simulink model "Z_Feedback_ROS"  (R2022b)
settings: Solver=FixedStepAuto  StartTime=0.0  StopTime=45  FixedStep=0.02  RelTol=1e-3
undefined symbols (not defined in the file): unicycle, X, Y
libraries: robotlib x3, simulink_extras x1
settings Model: Creator=mustacchim  LastModifiedBy=Musta
settings OptimizationCC: EnhancedBackFolding=on  PassReuseOutputArgsAs=Individual arguments  ZeroExternalMemoryAtStartup=off  ZeroInternalMemoryAtStartup=off  MaxStackSize=64  OptimizeBlockOrder=speed  DifferentSizesBufferReuse=on  OptimizationCustomize=off  EfficientTunableParamExpr=on
settings DebuggingCC: ParameterTunabilityLossMsg=error
settings HardwareCC: ProdBitPerPointer=32  ProdBitPerSizeT=32  ProdBitPerPtrDiffT=32  ProdLargestAtomicFloat=None  ProdIntDivRoundTo=Undefined  ProdEndianess=Unspecified  ProdWordSize=32  ProdHWDeviceType=Generic->Unspecified (assume 32-bit Generic)
settings SFSimCC: MATLABDynamicMemAlloc=off
settings RTWCC: Description=Embedded Coder  SystemTargetFile=ert.tlc  HardwareBoard=Robot Operating System (ROS)  TLCOptions="-aInlineSetEventsForThisBaseRateFcn=TLC_FALSE -aSuppressMultiTaskScheduler=TLC_FALSE  -aRateBasedStepFcn=0"  TemplateMakefile=ert_default_tmf  Toolchain=Catkin  TargetLang=C++
settings CodeAppCC: ForceParamTrailComments=on  IgnoreCustomStorageClasses=off  OperatorAnnotations=on  SimulinkDataObjDesc=on  SFDataObjDesc=on  InsertBlockDesc=on

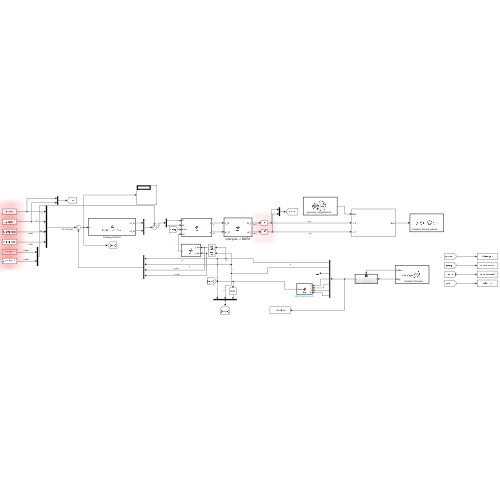
[thumbnail: Simulink's stored preview of the top-level diagram]
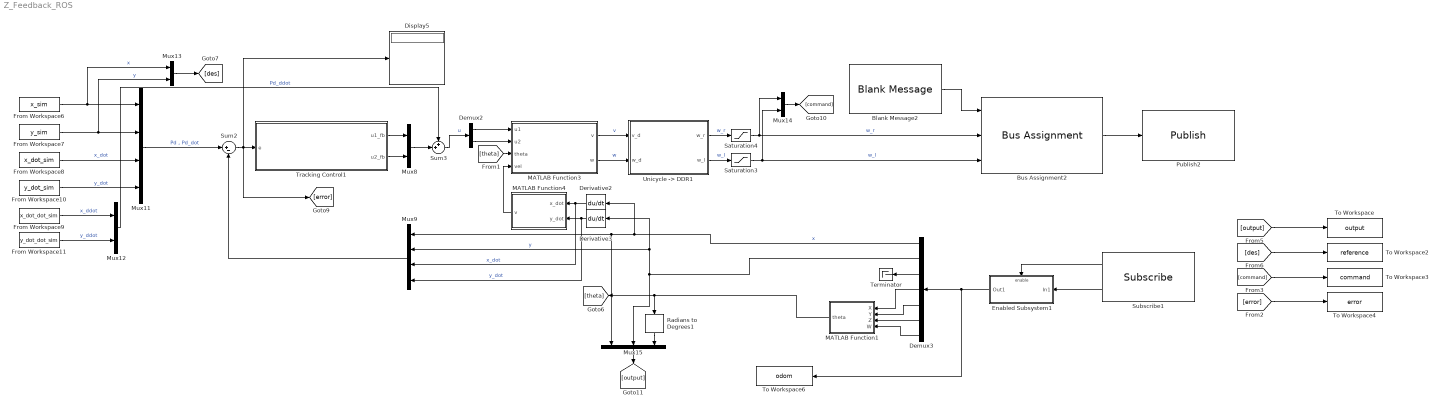
== system Z_Feedback_ROS ==
  Blank Message2 : robotlib/Blank Message  messageClass=Message  entityType=geometry_msgs/Vector3  messageType=geometry_msgs/Vector3  SampleTime=0.02  legacyBusStruct=off
      settings: LibrarySourceBlock=roslib/ROS/Blank Message
  Bus Assignment2 : BusAssignment  AssignedSignals=X,Y
  Demux2 : Demux  Outputs=2
  Demux3 : Demux  Outputs=7
  Derivative2 : Derivative
  Derivative3 : Derivative
  Display5 : Display
  Enabled Subsystem1 : Subsystem  TreatAsAtomicUnit=on
  From Workspace10 : FromWorkspace  VariableName=y_dot_sim
  From Workspace11 : FromWorkspace  VariableName=y_dot_dot_sim
  From Workspace6 : FromWorkspace  VariableName=x_sim
  From Workspace7 : FromWorkspace  VariableName=y_sim
  From Workspace8 : FromWorkspace  VariableName=x_dot_sim
  From Workspace9 : FromWorkspace  VariableName=x_dot_dot_sim
  MATLAB Function1 : MATLAB Function  TreatAsAtomicUnit=on
  MATLAB Function3 : MATLAB Function  TreatAsAtomicUnit=on
  MATLAB Function4 : MATLAB Function  TreatAsAtomicUnit=on
  Mux11 : Mux
  Mux{8,12..14} (4 alike) : Mux  Inputs=2
  Mux15 : Mux  Inputs=3
  Mux9 : Mux
  Publish2 : robotlib/Publish  topicSource=Select from ROS network  topic=/turtlebot_03/cmd_wheels  messageType=geometry_msgs/Vector3  legacyBusStruct=off  messageQueueLength=1
      settings: LibrarySourceBlock=roslib/ROS/Publish
  Radians to Degrees1 : simulink_extras/Transformations/Radians to Degrees
  Saturation3 : Saturate  UpperLimit=unicycle.omegaWheelMax  LowerLimit=unicycle.omegaWheelMin
  Saturation4 : Saturate  UpperLimit=unicycle.omegaWheelMax  LowerLimit=unicycle.omegaWheelMin
  Subscribe1 : robotlib/Subscribe  topicSource=Select from ROS network  topic=/turtlebot_03/odom  messageType=nav_msgs/Odometry  SampleTime=0.02  legacyBusStruct=off  messageQueueLength=1
      settings: LibrarySourceBlock=roslib/ROS/Subscribe
  Sum2 : Sum  Inputs=|+-
  Sum3 : Sum  Inputs=++|
  Terminator : Terminator
  To Workspace : ToWorkspace  VariableName=output  SaveFormat=Structure With Time  SampleTime=-1
  To Workspace2 : ToWorkspace  VariableName=reference  SaveFormat=Structure With Time  SampleTime=-1
  To Workspace3 : ToWorkspace  VariableName=command  SaveFormat=Structure With Time  SampleTime=-1
  To Workspace4 : ToWorkspace  VariableName=error  SaveFormat=Structure With Time  SampleTime=-1
  To Workspace6 : ToWorkspace  VariableName=odom  SaveFormat=Structure With Time  SampleTime=-1
  Tracking Control1 : MATLAB Function  TreatAsAtomicUnit=on
  "Unicycle -> DDR1" : MATLAB Function  TreatAsAtomicUnit=on
  wires:
  [command] -> To Workspace3/1
  [des] -> To Workspace2/1
  [error] -> To Workspace4/1
  [output] -> To Workspace/1
  From Workspace6/1 -> Mux13/1, Mux11/1  "x"
  Mux14/1 -> [command]
  MATLAB Function4/1(v) -> MATLAB Function3/4(vel)
  Mux9/1 -> Sum2/2
  Derivative2/1 -> Mux9/3, MATLAB Function4/1(x_dot)  "x_dot"
  MATLAB Function3/1(v) -> "Unicycle -> DDR1"/1(v_d)  "v"
  From Workspace8/1 -> Mux11/3  "x_dot"
  From Workspace10/1 -> Mux11/4  "y_dot"
  Bus Assignment2/1 -> Publish2/1
  Saturation3/1 -> Bus Assignment2/3, Mux14/2  "w_l"
  Tracking Control1/2(u2_fb) -> Mux8/2
  Blank Message2/1 -> Bus Assignment2/1
  From Workspace7/1 -> Mux13/2, Mux11/2  "y"
  Derivative3/1 -> Mux9/4, MATLAB Function4/2(y_dot)  "y_dot"
  Demux2/2 -> MATLAB Function3/2(u2)
  Saturation4/1 -> Bus Assignment2/2, Mux14/1  "w_r"
  "Unicycle -> DDR1"/1(w_r) -> Saturation4/1  "w_r"
  From Workspace11/1 -> Mux12/2  "y_ddot"
  MATLAB Function3/2(w) -> "Unicycle -> DDR1"/2(w_d)  "w"
  Mux12/1 -> Sum3/1  "Pd_ddot"
  [theta] -> MATLAB Function3/3(theta)
  "Unicycle -> DDR1"/2(w_l) -> Saturation3/1  "w_l"
  Mux13/1 -> [des]
  Mux11/1 -> Sum2/1  "Pd , Pd_dot"
  Demux2/1 -> MATLAB Function3/1(u1)
  Sum3/1 -> Demux2/1  "u"
  From Workspace9/1 -> Mux12/1  "x_ddot"
  Mux15/1 -> [output]
  Tracking Control1/1(u1_fb) -> Mux8/1
  Mux8/1 -> Sum3/2
  Sum2/1 -> Display5/1, [error], Tracking Control1/1(e)
  Radians to Degrees1/1 -> Mux15/3
  Enabled Subsystem1/1(Out1) -> Demux3/1, To Workspace6/1
  Subscribe1/1 -> Enabled Subsystem1/Enable
  Demux3/2 -> Mux9/2, Derivative3/1, Mux15/2  "y"
  Demux3/3 -> Terminator/1
  Subscribe1/2 -> Enabled Subsystem1/1(In1)
  Demux3/1 -> Mux9/1, Mux15/1, Derivative2/1  "x"
  MATLAB Function1/1(theta) -> [theta], Radians to Degrees1/1
  Demux3/5 -> MATLAB Function1/2(Y)
  Demux3/6 -> MATLAB Function1/3(Z)
  Demux3/4 -> MATLAB Function1/1(X)
  Demux3/7 -> MATLAB Function1/4(W)

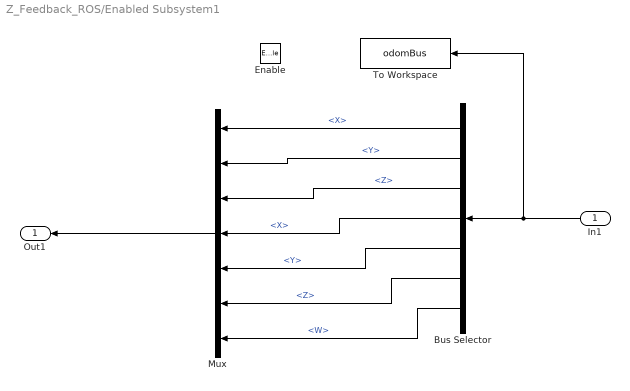
== system Z_Feedback_ROS/Enabled Subsystem1 ==
  In1 : Inport
  Enable : EnablePort
  Bus Selector : BusSelector  OutputSignals=Pose.Pose.Position.X,Pose.Pose.Position.Y,Pose.Pose.Position.Z,Pose.Pose.Orientation.X,Pose.Pose.Orientation.Y,Pose.Pose.Orientation.Z,Pose.Pose.Orientation.W
  Mux : Mux  Inputs=7
  To Workspace : ToWorkspace  VariableName=odomBus  SaveFormat=Timeseries  SampleTime=-1
  Out1 : Outport
  wires:
  Mux/1 -> Out1/1
  Bus Selector/1 -> Mux/1  "<X>"
  Bus Selector/2 -> Mux/2  "<Y>"
  In1/1 -> To Workspace/1, Bus Selector/1
  Bus Selector/3 -> Mux/3  "<Z>"
  Bus Selector/4 -> Mux/4  "<X>"
  Bus Selector/5 -> Mux/5  "<Y>"
  Bus Selector/6 -> Mux/6  "<Z>"
  Bus Selector/7 -> Mux/7  "<W>"

== matlab function Z_Feedback_ROS/MATLAB Function1 ==
  data: X input; theta output; Y input; Z input; W input
function theta = fcn(X, Y, Z, W)

    q_x = X;
    q_y = Y;
    q_z = Z;
    q_w = W;
    
    q = cat(2,q_x,q_y,q_z,q_w); 
    eulZYX = quat2eul(q,'ZYX');
    theta = eulZYX(:,3);
    
end

== matlab function Z_Feedback_ROS/MATLAB Function3 ==
  data: u1 input; u2 input; theta input; v output; w output; vel input
function [v,w] = T_inv(u1,u2,theta,vel)


if abs(vel) < 1e-3
    if abs(vel) >= 0
        vel = 1e-3;
    else 
        vel = -1e-3;
    end
end

T_i = [cos(theta) sin(theta);
      -sin(theta)/vel cos(theta)/vel];

v_w = T_i * [u1;u2];

v = v_w(1);
w = v_w(2);

== matlab function Z_Feedback_ROS/MATLAB Function4 ==
  data: x_dot input; v output; y_dot input
function v = vel(x_dot,y_dot)

v = sqrt(x_dot^2 + y_dot^2);

== matlab function Z_Feedback_ROS/Tracking Control1 ==
  data: u1_fb output; u2_fb output; e input
function [u1_fb,u2_fb] = tracking_controller(e)

    %#codegen
    coder.extrinsic('evalin')
    k_p1 = 0;                  % Needed in order to set variable class correctly
    k_p2 = 0;                  % Needed in order to set variable class correctly
    k_d1 = 0;                  % Needed in order to set variable class correctly
    k_d2 = 0;                  % Needed in order to set variable class correctly
    k_p1 = evalin('base','k_p1'); % Read value from workspace
    k_p2 = evalin('base','k_p2'); % Read value from workspace
    k_d1 = evalin('base','k_d1'); % Read value from workspace
    k_d2 = evalin('base','k_d2'); % Read value from workspace

    e_x = e(1);
    e_y = e(2);
    e_xdot = e(3);
    e_ydot = e(4);
    
    % Controller
    u1_fb = k_p1 * e_x + k_d1 * e_xdot;
    u2_fb = k_p2 *e_y + k_d2 * e_ydot;

end

== matlab function Z_Feedback_ROS/Unicycle -> DDR1 ==
  data: v_d input; w_r output; w_d input; w_l output
function [w_r, w_l] = fcn(v_d, w_d)

    %#codegen
    coder.extrinsic('evalin')
    d = 0;                  % Needed in order to set variable class correctly
    r = 0;                  % Needed in order to set variable class correctly
    d = evalin('base','unicycle.d'); % Read value from workspace
    r = evalin('base','unicycle.r'); % Read value from workspace

    w_r = ((2 * v_d) + (w_d * d)) / (2 * r);
    w_l = ((2 * v_d) - (w_d * d)) / (2 * r);

end
